simulink model "simulation42_25_10"  (R2019b)
settings: Solver=VariableStepAuto  StartTime=0.0  StopTime=10.0  RelTol=1e-3
settings Model: Creator=maxim  LastModifiedBy=maxim

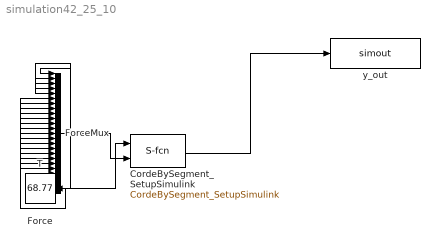
== system simulation42_25_10 ==
  CordeBySegment_SetupSimulink : M-S-Function  FunctionName=CordeBySegment_SetupSimulink  Parameters=3.250000e-03, 4.430000e-01, 0, 25, 1.000000e-04
  Force : Constant  Value=0
  ForceMux : Mux  Inputs=25
  T : Constant  Value=68.77
  y_out : ToWorkspace  VariableName=simout  SaveFormat=Timeseries  SampleTime=-1
  wires:
  Force/1 -> ForceMux/1, ForceMux/2, ForceMux/3, ForceMux/4, ForceMux/5, ForceMux/6, ForceMux/7, ForceMux/8, ForceMux/9, ForceMux/10, ForceMux/11, ForceMux/12, ForceMux/13, ForceMux/14, ForceMux/15, ForceMux/16, ForceMux/17, ForceMux/18, ForceMux/19, ForceMux/20, ForceMux/21, ForceMux/22, ForceMux/23, ForceMux/24, ForceMux/25
  T/1 -> CordeBySegment_SetupSimulink/1
  ForceMux/1 -> CordeBySegment_SetupSimulink/2
  CordeBySegment_SetupSimulink/1 -> y_out/1
